simulink model "Batch_Reactor_Simulation_Series_Reaction_A_B_C_Approach2"  (R2025a)
settings: Solver=FixedStepAuto  StartTime=0.0  StopTime=50  RelTol=1e-3
settings Model: Creator=must2  LastModifiedBy=must2

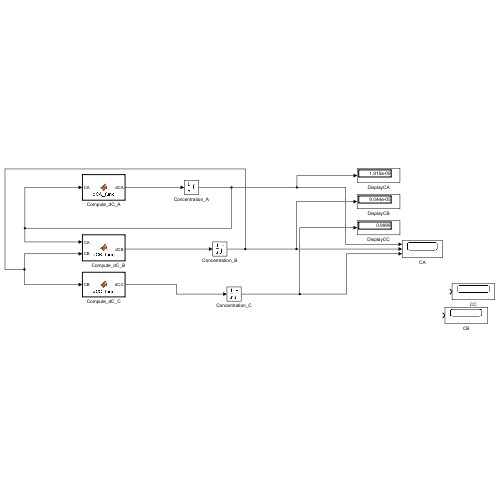
[thumbnail: Simulink's stored preview of the top-level diagram]
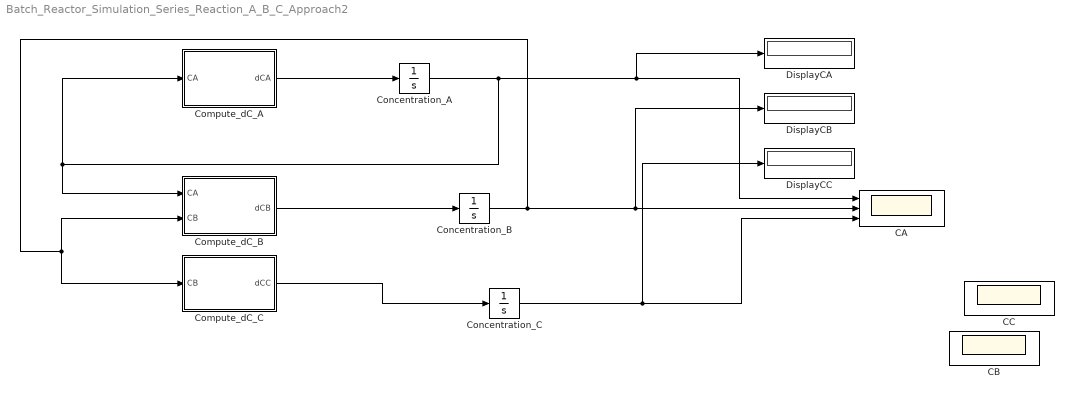
== system Batch_Reactor_Simulation_Series_Reaction_A_B_C_Approach2 ==
  "\tCompute_dC_B" : MATLAB Function  TreatAsAtomicUnit=on
  CA : Scope  NumInputPorts=3
      settings: Title=Batch Reactor Simulation: Concentration Profile of A --> B --> C Over Time  ActiveDisplayYMinimum=-0.1249999978458536  ActiveDisplayYMaximum=1.1249999997606503  YLabel=Concentration (mol/L)
  CB : Scope
      settings: Title=Batch Reactor Simulation: Concentration Profile of B Over Time  ActiveDisplayYMinimum=-0.062204169481481469  ActiveDisplayYMaximum=0.55983752533333331  YLabel=Concentration of B (mol/L)
  CC : Scope
      settings: Title=Batch Reactor Simulation: Concentration Profile of C Over Time  ActiveDisplayYMinimum=-0.15236578853621635  ActiveDisplayYMaximum=1.1600155046903078  YLabel=Concentration of C (mol/L)  DataLoggingVariableName=ScopeData2
  Compute_dC_A : MATLAB Function  TreatAsAtomicUnit=on
  Compute_dC_C : MATLAB Function  TreatAsAtomicUnit=on
  Concentration_A : Integrator  InitialCondition=5  LimitOutput=on  UpperSaturationLimit=1  LowerSaturationLimit=0
  Concentration_B : Integrator  LimitOutput=on  UpperSaturationLimit=1  LowerSaturationLimit=0
  Concentration_C : Integrator  LimitOutput=on  UpperSaturationLimit=1  LowerSaturationLimit=0
  DisplayCA : Display
  DisplayCB : Display
  DisplayCC : Display
  wires:
  Compute_dC_A/1(dCA) -> Concentration_A/1
  "\tCompute_dC_B"/1(dCB) -> Concentration_B/1
  Concentration_B/1 -> CA/2, DisplayCB/1, "\tCompute_dC_B"/2(CB), Compute_dC_C/1(CB)
  Concentration_A/1 -> Compute_dC_A/1(CA), "\tCompute_dC_B"/1(CA), CA/1, DisplayCA/1
  Compute_dC_C/1(dCC) -> Concentration_C/1
  Concentration_C/1 -> CA/3, DisplayCC/1

== matlab function Batch_Reactor_Simulation_Series_Reaction_A_B_C_Approach2/Compute_dC_A ==
  data: CA input; dCA output
function dCA = dCA_func(CA)
k1 = 0.4;
dCA = -k1 * CA;
end

== matlab function Batch_Reactor_Simulation_Series_Reaction_A_B_C_Approach2/Compute_dC_C ==
  data: CB input; dCC output
function dCC = dCC_func(CB)
k2 = 0.2;
dCC = k2 * CB;
end

== matlab function Batch_Reactor_Simulation_Series_Reaction_A_B_C_Approach2/	Compute_dC_B ==
  data: CA input; dCB output; CB input
function dCB = dCB_func(CA, CB)
k1 = 0.4;
k2 = 0.2;
dCB = k1 * CA - k2 * CB;
end
